simulink subsystem "HardwareOutputs"  (R2019b)
settings: Solver=VariableStepAuto  StartTime=0.0  StopTime=10.0  RelTol=1e-3
undefined symbols (not defined in the file): __PRM__SERIALIZED__DATA__, SubsystemReferenceBlock
settings Model: Creator=Nick  LastModifiedBy=Nick

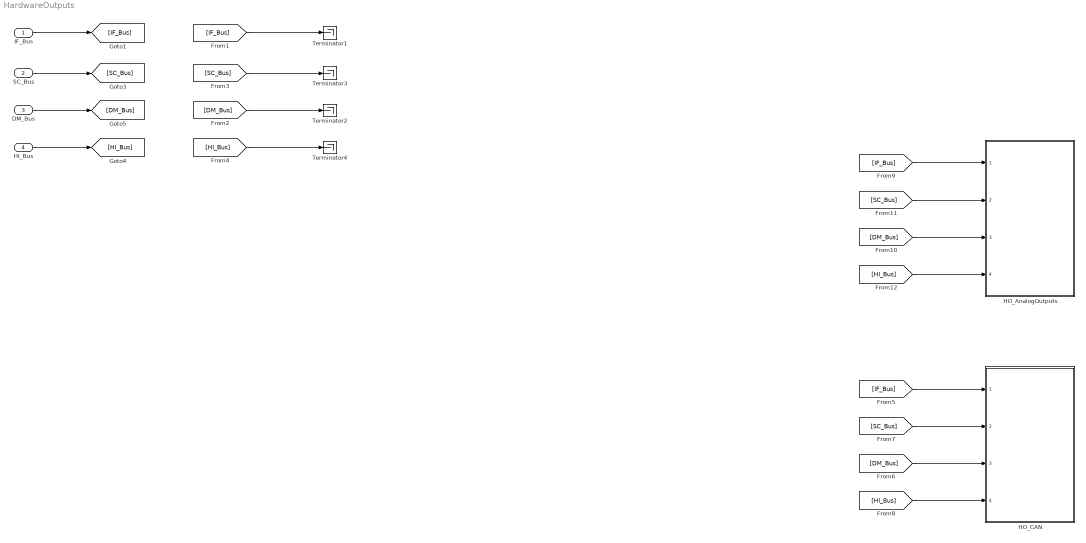
== system HardwareOutputs ==
  IF_Bus : Inport
  SC_Bus : Inport  Port=2
  DM_Bus : Inport  Port=3
  HI_Bus : Inport  Port=4
  HO_AnalogOutputs : Subsystem  BlockKeywords=__PRM__SERIALIZED__DATA__:SubsystemReferenceBlock  ReferencedSubsystem=HO_AnalogOutputs
  HO_CAN : Subsystem  BlockKeywords=__PRM__SERIALIZED__DATA__:SubsystemReferenceBlock  ReferencedSubsystem=HO_CAN
  Terminator{1..4} (4 alike) : Terminator
  wires:
  [SC_Bus] -> Terminator3/1
  SC_Bus/1 -> [SC_Bus]
  [IF_Bus] -> Terminator1/1
  HI_Bus/1 -> [HI_Bus]
  [HI_Bus] -> Terminator4/1
  IF_Bus/1 -> [IF_Bus]
  DM_Bus/1 -> [DM_Bus]
  [DM_Bus] -> Terminator2/1
  [IF_Bus] -> HO_CAN/1
  [DM_Bus] -> HO_CAN/3
  [HI_Bus] -> HO_CAN/4
  [SC_Bus] -> HO_CAN/2
  [SC_Bus] -> HO_AnalogOutputs/2
  [IF_Bus] -> HO_AnalogOutputs/1
  [HI_Bus] -> HO_AnalogOutputs/4
  [DM_Bus] -> HO_AnalogOutputs/3
